simulink model "model"  (R2019b)
settings: Solver=ode45  StartTime=0.0  StopTime=10  RelTol=1e-3
values from neighbouring files (symbols this model uses):
  K1 = 10    [de.m]    (also in initial_data.m)
  K3 = 1    [de.m]    (also in initial_data.m)
  K4 = 3    [de.m]    (also in initial_data.m)
  Kf = 0.2506628274631    (= 0.250662827463)    [de.m]    (also in initial_data.m)
  Klin = 0.11239753    [de.m]    (also in initial_data.m)
  T1 = 0.005    [de.m]    (also in initial_data.m)
  T3 = 0.05    [de.m]    (also in initial_data.m)
  T4 = 0.01    [de.m]    (also in initial_data.m)
  Tf = 0.1    [de.m]    (also in initial_data.m)
  v = 10    [de.m]    (also in initial_data.m)
  xi = 0.07    [de.m]    (also in initial_data.m)
libraries: simulink x1
settings Model: Creator=Roman  LastModifiedBy=Roman

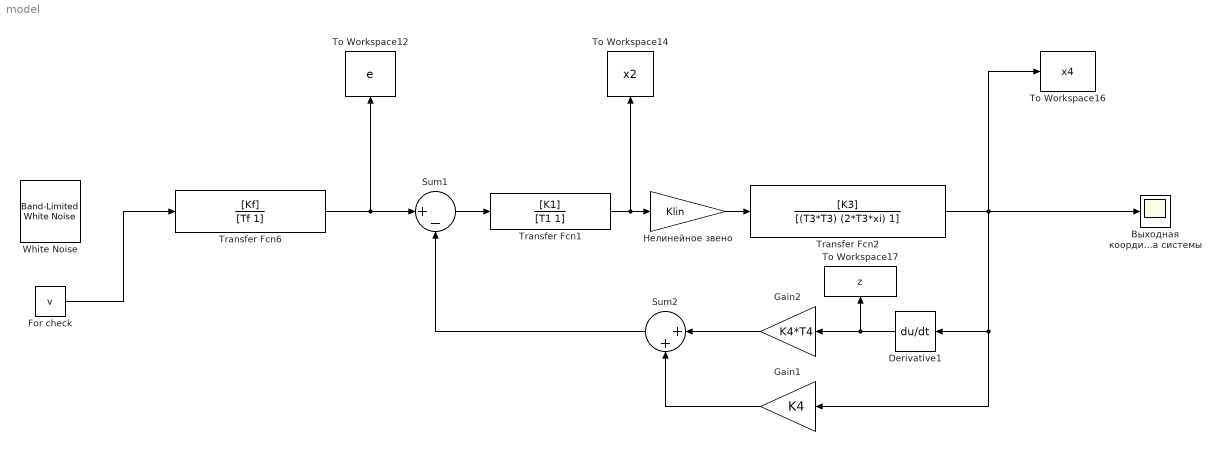
== system model ==
  Derivative1 : Derivative  CoefficientInTFapproximation=1
  "For check " : Constant  Value=v
  Gain1 : Gain  Gain=K4
  Gain2 : Gain  Gain=K4*T4
  Sum1 : Sum  Inputs=|+-
  Sum2 : Sum  Inputs=|++
  To Workspace12 : ToWorkspace  VariableName=e  SampleTime=-1
  To Workspace14 : ToWorkspace  VariableName=x2  SampleTime=-1
  To Workspace16 : ToWorkspace  VariableName=x4  SampleTime=-1
  To Workspace17 : ToWorkspace  VariableName=z  SampleTime=-1
  Transfer Fcn1 : TransferFcn  Numerator=[K1]  Denominator=[T1 1]
  Transfer Fcn2 : TransferFcn  Numerator=[K3]  Denominator=[(T3*T3) (2*T3*xi) 1]
  Transfer Fcn6 : TransferFcn  Numerator=[Kf]  Denominator=[Tf 1]
  White Noise : simulink/Sources/Band-Limited White Noise  Cov=[1]  Ts=0.0001  seed=100
  Выходная координата системы : Scope
  "Нелинейное звено " : Gain  Gain=Klin
  wires:
  Gain1/1 -> Sum2/2
  Transfer Fcn1/1 -> "Нелинейное звено "/1, To Workspace14/1
  Transfer Fcn6/1 -> Sum1/1, To Workspace12/1
  Transfer Fcn2/1 -> Gain1/1, Derivative1/1, To Workspace16/1, Выходная координата системы/1
  "Нелинейное звено "/1 -> Transfer Fcn2/1
  Sum2/1 -> Sum1/2
  Gain2/1 -> Sum2/1
  Sum1/1 -> Transfer Fcn1/1
  Derivative1/1 -> Gain2/1, To Workspace17/1
  "For check "/1 -> Transfer Fcn6/1
